simulink model "model_functie"  (R2017b)
settings: Solver=VariableStepAuto  StartTime=0.0  StopTime=10.0  RelTol=1e-3
settings Model: Creator=alinvoicu26  LastModifiedBy=alinvoicu26

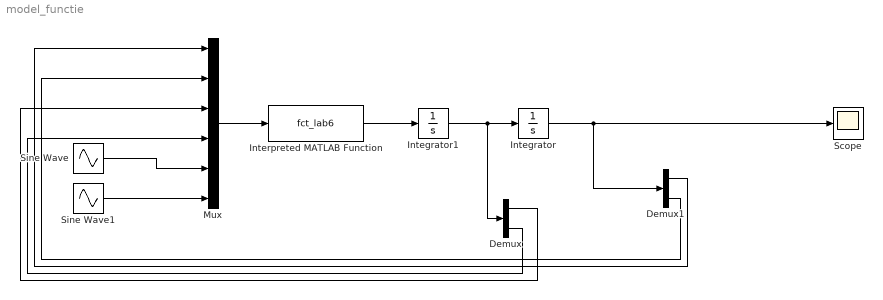
== system model_functie ==
  Demux : Demux  Outputs=2
  Demux1 : Demux  Outputs=2
  Integrator : Integrator
  Integrator1 : Integrator
  Interpreted MATLAB Function : MATLABFcn  MATLABFcn=fct_lab6  OutputDimensions=2
  Mux : Mux  Inputs=6
  Scope : Scope
  Sine Wave : Sin  SampleTime=0
  Sine Wave1 : Sin  SampleTime=0
  wires:
  Mux/1 -> Interpreted MATLAB Function/1
  Sine Wave1/1 -> Mux/6
  Sine Wave/1 -> Mux/5
  Interpreted MATLAB Function/1 -> Integrator1/1
  Integrator1/1 -> Demux/1, Integrator/1
  Integrator/1 -> Demux1/1, Scope/1
  Demux1/1 -> Mux/1
  Demux1/2 -> Mux/2
  Demux/1 -> Mux/3
  Demux/2 -> Mux/4
